simulink model "ModelPrediction"  (R2023b)
settings: Solver=VariableStepAuto  StartTime=0.0  StopTime=60  RelTol=1e-3
undefined symbols (not defined in the file): D1, D2, I
libraries: mcbcontrolslib x5, simulink x3
settings Model: Creator=markzhuang  LastModifiedBy=markzhuang

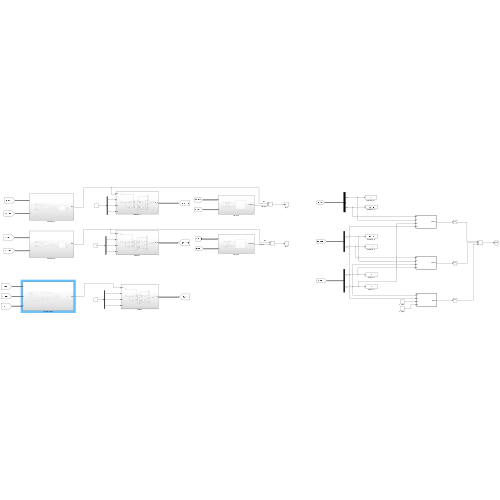
[thumbnail: Simulink's stored preview of the top-level diagram]
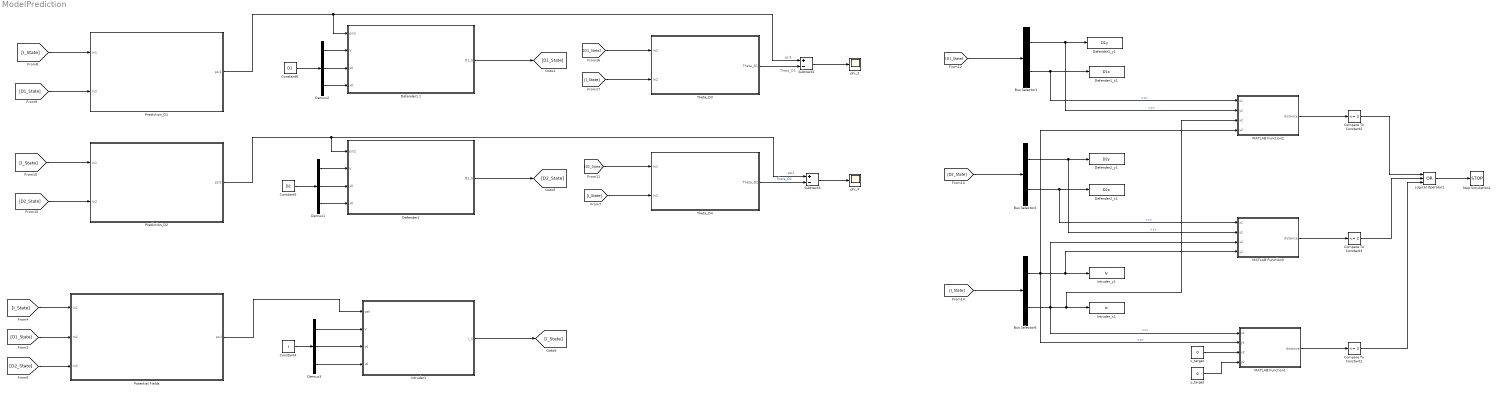
== system ModelPrediction ==
  note: Theta_D1
  note: psi2
  note: psi1
  Bus Selector1 : BusSelector  OutputSignals=y,x
  Bus Selector2 : BusSelector  OutputSignals=y,x
  Bus Selector6 : BusSelector  OutputSignals=y,x
  Compare To Constant1 : simulink/Logic and Bit Operations/Compare To Constant  relop=<=  const=2  OutDataTypeStr=boolean
  Compare To Constant2 : simulink/Logic and Bit Operations/Compare To Constant  relop=<=  const=2  OutDataTypeStr=boolean
  Compare To Constant3 : simulink/Logic and Bit Operations/Compare To Constant  relop=<=  const=2  OutDataTypeStr=boolean
  Constant4 : Constant  Value=I  VectorParams1D=off
  Constant5 : Constant  Value=D2  VectorParams1D=off
  Constant6 : Constant  Value=D1  VectorParams1D=off
  Defender1 : Subsystem
  Defender1 1 : Subsystem
  Defender1_x1 : ToWorkspace  VariableName=D1x  SaveFormat=Timeseries  SampleTime=-1
  Defender1_y1 : ToWorkspace  VariableName=D1y  SaveFormat=Timeseries  SampleTime=-1
  Defender2_x1 : ToWorkspace  VariableName=D2x  SaveFormat=Timeseries  SampleTime=-1
  Defender2_y1 : ToWorkspace  VariableName=D2y  SaveFormat=Timeseries  SampleTime=-1
  Demux1 : Demux  Outputs=3
  Demux2 : Demux  Outputs=3
  Demux5 : Demux  Outputs=3
  Intruder1 : Subsystem
  Intruder_x1 : ToWorkspace  VariableName=Ix  SaveFormat=Timeseries  SampleTime=-1
  Intruder_y1 : ToWorkspace  VariableName=Iy  SaveFormat=Timeseries  SampleTime=-1
  Logical Operator1 : Logic  Operator=OR  Inputs=3  AllPortsSameDT=off  OutDataTypeStr=boolean
  MATLAB Function1 : MATLAB Function  TreatAsAtomicUnit=on
  MATLAB Function2 : MATLAB Function  TreatAsAtomicUnit=on
  MATLAB Function3 : MATLAB Function  TreatAsAtomicUnit=on
  Potential Fields : Subsystem
  Prediction_D1 : Subsystem
  Prediction_D2 : Subsystem
  Stop Simulation1 : Stop
  Subtract2 : Sum  Inputs=+-
  Subtract3 : Sum  Inputs=+-
  Theta_D3 : Subsystem
  Theta_D4 : Subsystem
  phi_3 : Scope
  phi_4 : Scope
  x_target : Constant  Value=0
  y_target : Constant  Value=0
  wires:
  [I_State] -> Prediction_D1/1(In1)
  [I_State] -> Prediction_D2/1(In1)
  [D2_State] -> Prediction_D2/2(In2)
  [D1_State] -> Prediction_D1/2(In2)
  Logical Operator1/1 -> Stop Simulation1/1
  Constant5/1 -> Demux1/1
  Bus Selector6/1 -> MATLAB Function1/2(y1), MATLAB Function2/4(y2), MATLAB Function3/4(y2), Intruder_y1/1  "<y>"
  y_target/1 -> MATLAB Function1/4(y2)
  Demux5/2 -> Intruder1/3(y0)
  [D2_State] -> Potential Fields/3(In3)
  [I_State] -> Theta_D3/2(In2)
  Demux5/3 -> Intruder1/4(x0)
  Bus Selector2/1 -> MATLAB Function3/2(y1), Defender2_y1/1  "<y>"
  [D1_State] -> Theta_D3/1(In1)
  Bus Selector6/2 -> MATLAB Function1/1(x1), MATLAB Function3/3(x2), MATLAB Function2/3(x2), Intruder_x1/1  "<x>"
  [I_State] -> Bus Selector6/1
  Defender1 1/1(D1_S) -> [D1_State]
  Constant6/1 -> Demux2/1
  Compare To Constant3/1 -> Logical Operator1/2
  Bus Selector2/2 -> MATLAB Function3/1(x1), Defender2_x1/1  "<x>"
  [D2_State] -> Bus Selector2/1
  [D1_State] -> Potential Fields/2(In2)
  Potential Fields/1(psiI) -> Intruder1/1(psiI)
  Defender1/1(D2_S) -> [D2_State]
  Bus Selector1/2 -> MATLAB Function2/1(x1), Defender1_x1/1  "<x>"
  x_target/1 -> MATLAB Function1/3(x2)
  Compare To Constant1/1 -> Logical Operator1/3
  Demux5/1 -> Intruder1/2(V)
  [D1_State] -> Bus Selector1/1
  MATLAB Function2/1(distance) -> Compare To Constant2/1
  Theta_D3/1(Theta_D1) -> Subtract2/2
  Subtract2/1 -> phi_3/1
  [I_State] -> Theta_D4/2(In2)
  [D2_State] -> Theta_D4/1(In1)
  Compare To Constant2/1 -> Logical Operator1/1
  Intruder1/1(I_S) -> [I_State]
  [I_State] -> Potential Fields/1(In1)
  MATLAB Function1/1(distance) -> Compare To Constant1/1
  Theta_D4/1(Theta_D2) -> Subtract3/2  "Theta_D2"
  Bus Selector1/1 -> MATLAB Function2/2(y1), Defender1_y1/1  "<y>"
  Constant4/1 -> Demux5/1
  MATLAB Function3/1(distance) -> Compare To Constant3/1
  Subtract3/1 -> phi_4/1
  Prediction_D1/1(psi1) -> Defender1 1/1(psi1), Subtract2/1
  Prediction_D2/1(psi2) -> Subtract3/1, Defender1/1(psi2)
  Demux1/3 -> Defender1/4(x0)
  Demux1/2 -> Defender1/3(y0)
  Demux1/1 -> Defender1/2(V)
  Demux2/3 -> Defender1 1/4(x0)
  Demux2/2 -> Defender1 1/3(y0)
  Demux2/1 -> Defender1 1/2(V)

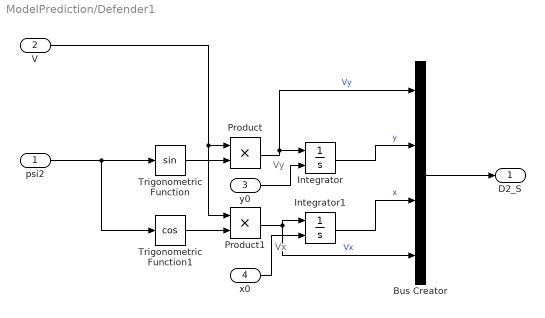
== system ModelPrediction/Defender1 ==
  note: Vx
  note: Vy
  psi2 : Inport
  V : Inport  Port=2
  y0 : Inport  Port=3
  x0 : Inport  Port=4
  Bus Creator : BusCreator  Inputs=4
  Integrator : Integrator  InitialConditionSource=external
  Integrator1 : Integrator  InitialConditionSource=external
  Product : Product
  Product1 : Product
  Trigonometric Function : Trigonometry
  Trigonometric Function1 : Trigonometry  Operator=cos
  D2_S : Outport
  wires:
  Trigonometric Function/1 -> Product/2
  Product/1 -> Bus Creator/1, Integrator/1  "Vy"
  psi2/1 -> Trigonometric Function1/1, Trigonometric Function/1
  Product1/1 -> Bus Creator/4, Integrator1/1  "Vx"
  V/1 -> Product1/1, Product/1
  Trigonometric Function1/1 -> Product1/2
  Integrator/1 -> Bus Creator/2  "y"
  Integrator1/1 -> Bus Creator/3  "x"
  y0/1 -> Integrator/2
  x0/1 -> Integrator1/2
  Bus Creator/1 -> D2_S/1

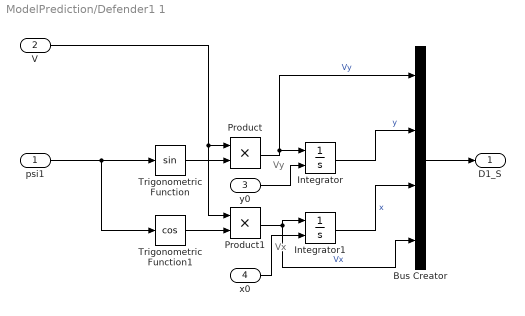
== system ModelPrediction/Defender1 1 ==
  note: Vx
  note: Vy
  psi1 : Inport
  V : Inport  Port=2
  y0 : Inport  Port=3
  x0 : Inport  Port=4
  Bus Creator : BusCreator  Inputs=4
  Integrator : Integrator  InitialConditionSource=external
  Integrator1 : Integrator  InitialConditionSource=external
  Product : Product
  Product1 : Product
  Trigonometric Function : Trigonometry
  Trigonometric Function1 : Trigonometry  Operator=cos
  D1_S : Outport
  wires:
  Trigonometric Function/1 -> Product/2
  psi1/1 -> Trigonometric Function1/1, Trigonometric Function/1
  Product1/1 -> Bus Creator/4, Integrator1/1  "Vx"
  V/1 -> Product1/1, Product/1
  Trigonometric Function1/1 -> Product1/2
  y0/1 -> Integrator/2
  x0/1 -> Integrator1/2
  Product/1 -> Bus Creator/1, Integrator/1  "Vy"
  Integrator/1 -> Bus Creator/2  "y"
  Integrator1/1 -> Bus Creator/3  "x"
  Bus Creator/1 -> D1_S/1

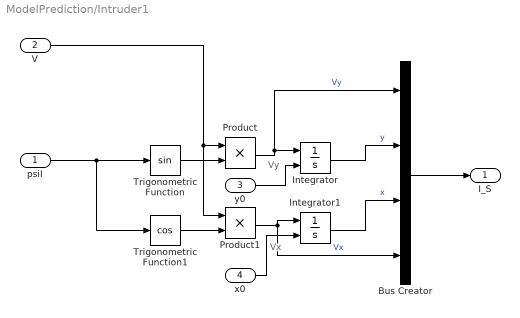
== system ModelPrediction/Intruder1 ==
  note: Vx
  note: Vy
  psiI : Inport
  V : Inport  Port=2
  y0 : Inport  Port=3
  x0 : Inport  Port=4
  Bus Creator : BusCreator  Inputs=4
  Integrator : Integrator  InitialConditionSource=external
  Integrator1 : Integrator  InitialConditionSource=external
  Product : Product
  Product1 : Product
  Trigonometric Function : Trigonometry
  Trigonometric Function1 : Trigonometry  Operator=cos
  I_S : Outport
  wires:
  Trigonometric Function/1 -> Product/2
  Product/1 -> Bus Creator/1, Integrator/1  "Vy"
  psiI/1 -> Trigonometric Function1/1, Trigonometric Function/1
  Product1/1 -> Bus Creator/4, Integrator1/1  "Vx"
  V/1 -> Product1/1, Product/1
  Trigonometric Function1/1 -> Product1/2
  Integrator/1 -> Bus Creator/2  "y"
  Integrator1/1 -> Bus Creator/3  "x"
  y0/1 -> Integrator/2
  x0/1 -> Integrator1/2
  Bus Creator/1 -> I_S/1

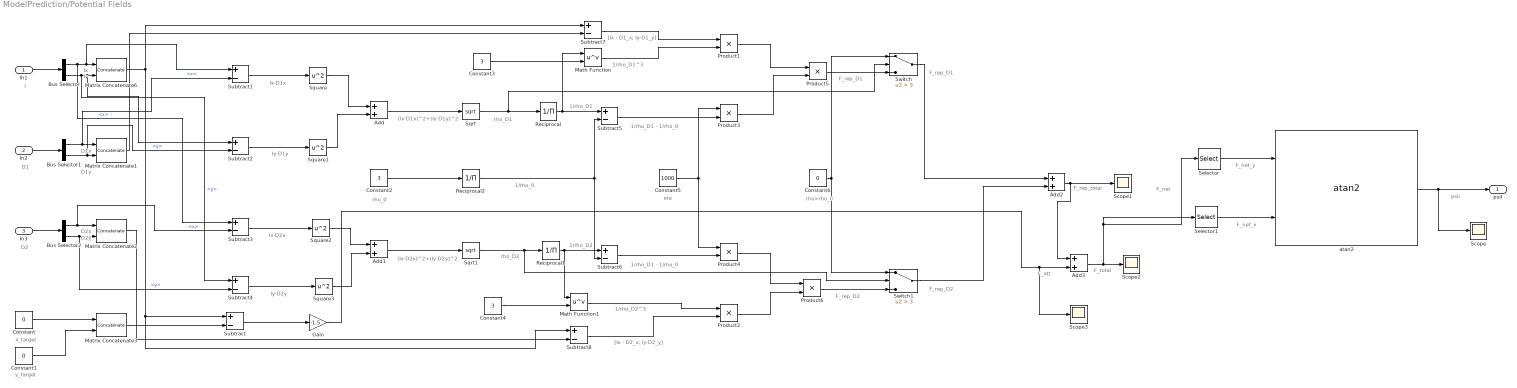
== system ModelPrediction/Potential Fields ==
  note: F_total
  note: psil
  note: F_net_y
  note: F_net
  note: F_rep_total
  note: rho>rho_0
  note: F_rep_D1
  note: eta
  note: [Ix - D2_x; Iy-D2_y]
  note: [Ix - D1_x; Iy-D1_y]
  note: 1/rho_D1^3
  note: 1/rho_0
  note: rho_0
  note: rho_D2
  note: rho_D1
  note: (Ix-D2x)^2+(Iy-D2y)^2
  note: (Ix-D1x)^2+(Iy-D1y)^2
  note: Iy-D2y
  note: Ix-D2x
  note: Ix-D1x
  note: Iy-D1y
  note: F_att
  note: x_target
  note: y_target
  note: D2x
  note: D2y
  note: D1x
  note: D1y
  note: Ix
  note: Iy
  note: D2
  note: I
  note: D1
  note: 1/rho_D1
  note: 1/rho_D2
  note: 1/rho_D1 - 1/rho_0
  note: 1/rho_D1 - 1/rho_0
  note: 1/rho_D2^3
  note: F_rep_D2
  note: F_rep_D1
  note: F_rep_D2
  note: F_net_x
  In1 : Inport
  In2 : Inport  Port=2
  In3 : Inport  Port=3
  Add{,1..3} (4 alike) : Sum
  Bus Selector : BusSelector  OutputSignals=x,y
  Bus Selector1 : BusSelector  OutputSignals=x,y
  Bus Selector2 : BusSelector  OutputSignals=x,y
  Constant : Constant  Value=0
  Constant1 : Constant  Value=0
  Constant2 : Constant  Value=3
  Constant3 : Constant  Value=3
  Constant4 : Constant  Value=3
  Constant5 : Constant  Value=1000
  Constant6 : Constant  Value=0
  Gain : Gain  Gain=-1.5
  Math Function : Math  Operator=pow
  Math Function1 : Math  Operator=pow
  Matrix Concatenate{1..3,6} (4 alike) : Concatenate  Mode=Multidimensional array
  Product{1..6} (6 alike) : Product
  Reciprocal : Product  Inputs=/
  Reciprocal1 : Product  Inputs=/
  Reciprocal2 : Product  Inputs=/
  Scope{,1..3} (4 alike) : Scope
  Selector : Selector  InputPortWidth=2  IndexOptions=Index vector (dialog)  Indices=2  OutputSizes=1
  Selector1 : Selector  InputPortWidth=2  IndexOptions=Index vector (dialog)  Indices=1  OutputSizes=1
  Sqrt : Sqrt
  Sqrt1 : Sqrt
  Square{,1..3} (4 alike) : Math  Operator=square
  Subtract{,1..8} (9 alike) : Sum  Inputs=+-
  Switch : Switch  Criteria=u2 > Threshold  Threshold=3  SaturateOnIntegerOverflow=off  InputSameDT=off
  Switch1 : Switch  Criteria=u2 > Threshold  Threshold=3  SaturateOnIntegerOverflow=off  InputSameDT=off
  atan2 : mcbcontrolslib/atan2  ApproximationMethod=None  NumberOfIterations=11  NumberOfDataPoints=16  InterpMethod=Flat  outputUnit=Radians  TableDataTypeStr=Inherit: Inherit via input
      settings: LibrarySourceBlock=mcblib/Controls/Math Transforms/atan2
  psiI : Outport
  wires:
  In1/1 -> Bus Selector/1
  In2/1 -> Bus Selector1/1
  In3/1 -> Bus Selector2/1
  Constant/1 -> Matrix Concatenate3/1
  Constant1/1 -> Matrix Concatenate3/2
  Matrix Concatenate3/1 -> Subtract/2
  Subtract/1 -> Gain/1
  Subtract1/1 -> Square/1
  Subtract2/1 -> Square1/1
  Subtract3/1 -> Square2/1
  Subtract4/1 -> Square3/1
  Square/1 -> Add/1
  Square1/1 -> Add/2
  Square2/1 -> Add1/1
  Square3/1 -> Add1/2
  Add/1 -> Sqrt/1
  Add1/1 -> Sqrt1/1
  Sqrt/1 -> Switch/2, Reciprocal/1
  Sqrt1/1 -> Switch1/2, Reciprocal1/1
  Reciprocal/1 -> Math Function/1, Subtract5/1
  Constant2/1 -> Reciprocal2/1
  Reciprocal2/1 -> Subtract5/2, Subtract6/2
  Reciprocal1/1 -> Math Function1/1, Subtract6/1
  Subtract5/1 -> Product3/2
  Subtract6/1 -> Product4/2
  Constant3/1 -> Math Function/2
  Constant4/1 -> Math Function1/2
  Math Function/1 -> Product1/2
  Math Function1/1 -> Product2/1
  Bus Selector/1 -> Subtract3/1, Subtract1/1, Matrix Concatenate6/1  "<x>"
  Bus Selector/2 -> Subtract4/1, Subtract2/1, Matrix Concatenate6/2  "<y>"
  Bus Selector1/1 -> Subtract1/2, Matrix Concatenate1/1  "<x>"
  Bus Selector1/2 -> Subtract2/2, Matrix Concatenate1/2  "<y>"
  Bus Selector2/1 -> Subtract3/2, Matrix Concatenate2/1  "<x>"
  Bus Selector2/2 -> Subtract4/2, Matrix Concatenate2/2  "<y>"
  Matrix Concatenate6/1 -> Subtract8/1, Subtract/1, Subtract7/1
  Matrix Concatenate1/1 -> Subtract7/2
  Matrix Concatenate2/1 -> Subtract8/2
  Subtract7/1 -> Product1/1
  Subtract8/1 -> Product2/2
  Constant5/1 -> Product3/1, Product4/1
  Product1/1 -> Product5/1
  Product3/1 -> Product5/2
  Product4/1 -> Product6/1
  Product2/1 -> Product6/2
  Product6/1 -> Switch1/3
  Product5/1 -> Switch/3
  Constant6/1 -> Switch/1, Switch1/1
  Switch/1 -> Add2/1
  Switch1/1 -> Add2/2
  Selector1/1 -> atan2/2
  Selector/1 -> atan2/1
  atan2/1 -> Scope/1, psiI/1
  Add2/1 -> Add3/1, Scope1/1
  Gain/1 -> Scope3/1, Add3/2
  Add3/1 -> Selector1/1, Selector/1, Scope2/1

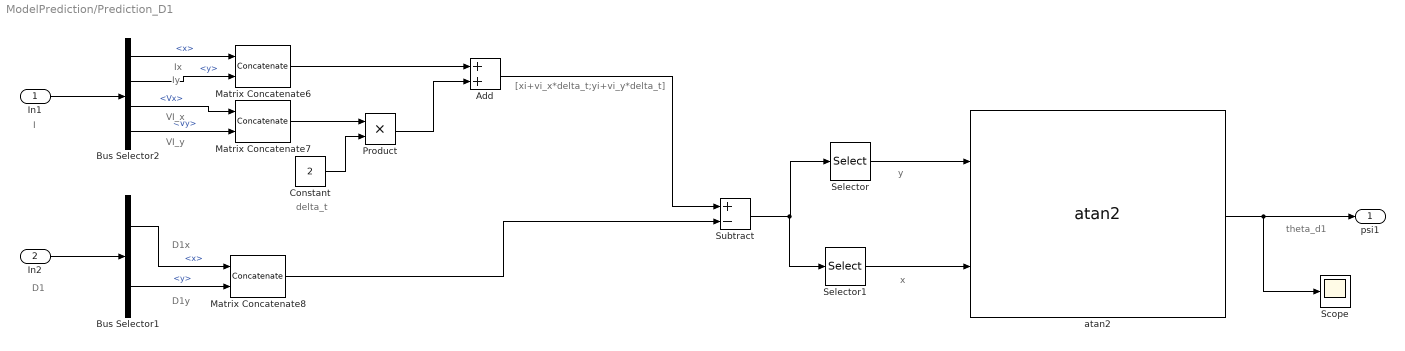
== system ModelPrediction/Prediction_D1 ==
  note: [xi+vi_x*delta_t;yi+vi_y*delta_t]
  note: delta_t
  note: D1
  note: I
  note: Iy
  note: Ix
  note: D1y
  note: D1x
  note: VI_y
  note: VI_x
  note: x
  note: y
  note: theta_d1
  In1 : Inport
  In2 : Inport  Port=2
  Add : Sum
  Bus Selector1 : BusSelector  OutputSignals=x,y
  Bus Selector2 : BusSelector  OutputSignals=x,y,Vx,Vy
  Constant : Constant  Value=2
  Matrix Concatenate6 : Concatenate  Mode=Multidimensional array
  Matrix Concatenate7 : Concatenate  Mode=Multidimensional array
  Matrix Concatenate8 : Concatenate  Mode=Multidimensional array
  Product : Product
  Scope : Scope
  Selector : Selector  InputPortWidth=2  IndexOptions=Index vector (dialog)  Indices=2  OutputSizes=1
  Selector1 : Selector  InputPortWidth=2  IndexOptions=Index vector (dialog)  Indices=1  OutputSizes=1
  Subtract : Sum  Inputs=+-
  atan2 : mcbcontrolslib/atan2  ApproximationMethod=None  NumberOfIterations=11  NumberOfDataPoints=16  InterpMethod=Flat  outputUnit=Radians  TableDataTypeStr=Inherit: Inherit via input
      settings: LibrarySourceBlock=mcblib/Controls/Math Transforms/atan2
  psi1 : Outport
  wires:
  In1/1 -> Bus Selector2/1
  In2/1 -> Bus Selector1/1
  Bus Selector2/4 -> Matrix Concatenate7/2  "<Vy>"
  Bus Selector2/1 -> Matrix Concatenate6/1  "<x>"
  Bus Selector1/2 -> Matrix Concatenate8/2  "<y>"
  Bus Selector2/3 -> Matrix Concatenate7/1  "<Vx>"
  Bus Selector1/1 -> Matrix Concatenate8/1  "<x>"
  Bus Selector2/2 -> Matrix Concatenate6/2  "<y>"
  Matrix Concatenate6/1 -> Add/1
  Matrix Concatenate7/1 -> Product/1
  Constant/1 -> Product/2
  Product/1 -> Add/2
  Add/1 -> Subtract/1
  Matrix Concatenate8/1 -> Subtract/2
  Selector1/1 -> atan2/2
  Selector/1 -> atan2/1
  atan2/1 -> Scope/1, psi1/1
  Subtract/1 -> Selector1/1, Selector/1

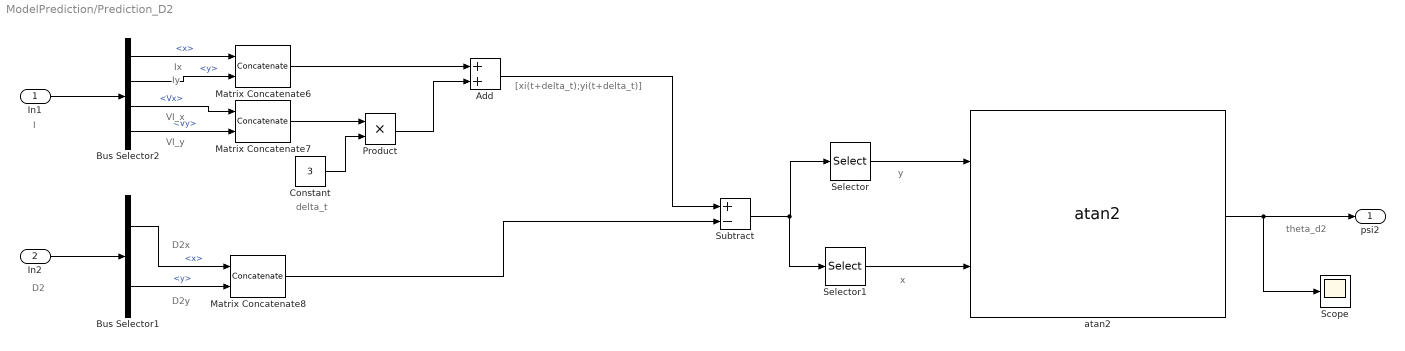
== system ModelPrediction/Prediction_D2 ==
  note: [xi(t+delta_t);yi(t+delta_t)]
  note: delta_t
  note: D2
  note: I
  note: Iy
  note: Ix
  note: D2y
  note: D2x
  note: VI_y
  note: VI_x
  note: x
  note: y
  note: theta_d2
  In1 : Inport
  In2 : Inport  Port=2
  Add : Sum
  Bus Selector1 : BusSelector  OutputSignals=x,y
  Bus Selector2 : BusSelector  OutputSignals=x,y,Vx,Vy
  Constant : Constant  Value=3
  Matrix Concatenate6 : Concatenate  Mode=Multidimensional array
  Matrix Concatenate7 : Concatenate  Mode=Multidimensional array
  Matrix Concatenate8 : Concatenate  Mode=Multidimensional array
  Product : Product
  Scope : Scope
  Selector : Selector  InputPortWidth=2  IndexOptions=Index vector (dialog)  Indices=2  OutputSizes=1
  Selector1 : Selector  InputPortWidth=2  IndexOptions=Index vector (dialog)  Indices=1  OutputSizes=1
  Subtract : Sum  Inputs=+-
  atan2 : mcbcontrolslib/atan2  ApproximationMethod=None  NumberOfIterations=11  NumberOfDataPoints=16  InterpMethod=Flat  outputUnit=Radians  TableDataTypeStr=Inherit: Inherit via input
      settings: LibrarySourceBlock=mcblib/Controls/Math Transforms/atan2
  psi2 : Outport
  wires:
  In1/1 -> Bus Selector2/1
  In2/1 -> Bus Selector1/1
  Bus Selector2/4 -> Matrix Concatenate7/2  "<Vy>"
  Bus Selector2/1 -> Matrix Concatenate6/1  "<x>"
  Bus Selector1/2 -> Matrix Concatenate8/2  "<y>"
  Bus Selector2/3 -> Matrix Concatenate7/1  "<Vx>"
  Bus Selector1/1 -> Matrix Concatenate8/1  "<x>"
  Bus Selector2/2 -> Matrix Concatenate6/2  "<y>"
  Matrix Concatenate6/1 -> Add/1
  Matrix Concatenate7/1 -> Product/1
  Constant/1 -> Product/2
  Product/1 -> Add/2
  Add/1 -> Subtract/1
  Matrix Concatenate8/1 -> Subtract/2
  Selector1/1 -> atan2/2
  Selector/1 -> atan2/1
  atan2/1 -> Scope/1, psi2/1
  Subtract/1 -> Selector1/1, Selector/1

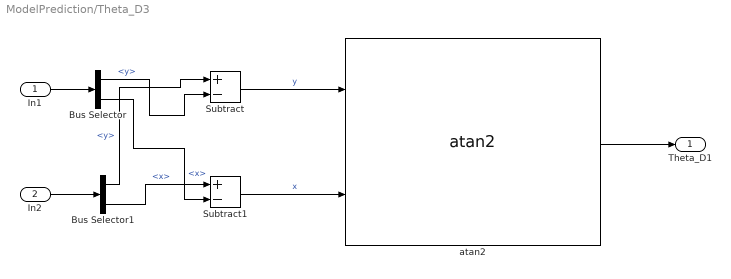
== system ModelPrediction/Theta_D3 ==
  In1 : Inport
  In2 : Inport  Port=2
  Bus Selector : BusSelector  OutputSignals=y,x
  Bus Selector1 : BusSelector  OutputSignals=y,x
  Subtract : Sum  Inputs=+-
  Subtract1 : Sum  Inputs=+-
  atan2 : mcbcontrolslib/atan2  ApproximationMethod=None  NumberOfIterations=11  NumberOfDataPoints=16  InterpMethod=Flat  outputUnit=Radians  TableDataTypeStr=Inherit: Inherit via input
      settings: LibrarySourceBlock=mcblib/Controls/Math Transforms/atan2
  Theta_D1 : Outport
  wires:
  In1/1 -> Bus Selector/1
  In2/1 -> Bus Selector1/1
  Bus Selector1/1 -> Subtract/1  "<y>"
  Bus Selector/1 -> Subtract/2  "<y>"
  Bus Selector1/2 -> Subtract1/1  "<x>"
  Bus Selector/2 -> Subtract1/2  "<x>"
  Subtract/1 -> atan2/1  "y"
  Subtract1/1 -> atan2/2  "x"
  atan2/1 -> Theta_D1/1

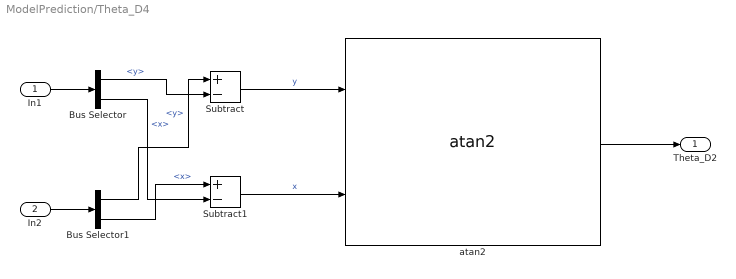
== system ModelPrediction/Theta_D4 ==
  In1 : Inport
  In2 : Inport  Port=2
  Bus Selector : BusSelector  OutputSignals=y,x
  Bus Selector1 : BusSelector  OutputSignals=y,x
  Subtract : Sum  Inputs=+-
  Subtract1 : Sum  Inputs=+-
  atan2 : mcbcontrolslib/atan2  ApproximationMethod=None  NumberOfIterations=11  NumberOfDataPoints=16  InterpMethod=Flat  outputUnit=Radians  TableDataTypeStr=Inherit: Inherit via input
      settings: LibrarySourceBlock=mcblib/Controls/Math Transforms/atan2
  Theta_D2 : Outport
  wires:
  In1/1 -> Bus Selector/1
  In2/1 -> Bus Selector1/1
  Bus Selector1/1 -> Subtract/1  "<y>"
  Bus Selector/1 -> Subtract/2  "<y>"
  Bus Selector1/2 -> Subtract1/1  "<x>"
  Bus Selector/2 -> Subtract1/2  "<x>"
  Subtract/1 -> atan2/1  "y"
  Subtract1/1 -> atan2/2  "x"
  atan2/1 -> Theta_D2/1

== matlab function ModelPrediction/MATLAB Function1 ==
  data: x1 input; distance output; y1 input; x2 input; y2 input
function distance = calculateDistance(x1, y1, x2, y2)
    distance = sqrt((x2 - x1)^2 + (y2 - y1)^2);
end

== matlab function ModelPrediction/MATLAB Function2 ==
  data: x1 input; distance output; y1 input; x2 input; y2 input
function distance = calculateDistance(x1, y1, x2, y2)
    distance = sqrt((x2 - x1)^2 + (y2 - y1)^2);
end

== matlab function ModelPrediction/MATLAB Function3 ==
  data: x1 input; distance output; y1 input; x2 input; y2 input
function distance = calculateDistance(x1, y1, x2, y2)
    distance = sqrt((x2 - x1)^2 + (y2 - y1)^2);
end
